simulink model "state_machine"  (R2017b)
settings: Solver=FixedStepAuto  StartTime=0.0  StopTime=1000  FixedStep=0.01  RelTol=1e-3
model workspace (MAT data in the model file):
  SL_ROS_VariableLengthArrays_MaxSizes.CommonInfo.ArrayTruncateAction = 'EmitWarning'
  SL_ROS_VariableLengthArrays_MaxSizes.MsgTypeMap = containers.Map
  SL_ROS_VariableLengthArrays_MaxSizes.MsgTypeMap.serialization.keys = {'sensor_msgs/JointState', 'trajectory_msgs/JointTrajectory', 'trajectory_msgs/JointTrajectoryPoint'}
  SL_ROS_VariableLengthArrays_MaxSizes.MsgTypeMap.serialization.values{1}(1).PropertyName = 'Effort'
  SL_ROS_VariableLengthArrays_MaxSizes.MsgTypeMap.serialization.values{1}(1).DataType = 'double'
  SL_ROS_VariableLengthArrays_MaxSizes.MsgTypeMap.serialization.values{1}(1).MaxLength = 7
  SL_ROS_VariableLengthArrays_MaxSizes.MsgTypeMap.serialization.values{1}(2).PropertyName = 'Name'
  SL_ROS_VariableLengthArrays_MaxSizes.MsgTypeMap.serialization.values{1}(2).DataType = 'std_msgs/String'
  SL_ROS_VariableLengthArrays_MaxSizes.MsgTypeMap.serialization.values{1}(2).MaxLength = 7
  SL_ROS_VariableLengthArrays_MaxSizes.MsgTypeMap.serialization.values{1}(3).PropertyName = 'Position'
  SL_ROS_VariableLengthArrays_MaxSizes.MsgTypeMap.serialization.values{1}(3).DataType = 'double'
  SL_ROS_VariableLengthArrays_MaxSizes.MsgTypeMap.serialization.values{1}(3).MaxLength = 7
  SL_ROS_VariableLengthArrays_MaxSizes.MsgTypeMap.serialization.values{1}(4).PropertyName = 'Velocity'
  SL_ROS_VariableLengthArrays_MaxSizes.MsgTypeMap.serialization.values{1}(4).DataType = 'double'
  SL_ROS_VariableLengthArrays_MaxSizes.MsgTypeMap.serialization.values{1}(4).MaxLength = 7
  SL_ROS_VariableLengthArrays_MaxSizes.MsgTypeMap.serialization.values{2}(1).PropertyName = 'JointNames'
  SL_ROS_VariableLengthArrays_MaxSizes.MsgTypeMap.serialization.values{2}(1).DataType = 'std_msgs/String'
  SL_ROS_VariableLengthArrays_MaxSizes.MsgTypeMap.serialization.values{2}(1).MaxLength = 7
  SL_ROS_VariableLengthArrays_MaxSizes.MsgTypeMap.serialization.values{2}(2).PropertyName = 'Points'
  SL_ROS_VariableLengthArrays_MaxSizes.MsgTypeMap.serialization.values{2}(2).DataType = 'trajectory_msgs/JointTrajectoryPoint'
  SL_ROS_VariableLengthArrays_MaxSizes.MsgTypeMap.serialization.values{2}(2).MaxLength = 1
  SL_ROS_VariableLengthArrays_MaxSizes.MsgTypeMap.serialization.values{3}(1).PropertyName = 'Accelerations'
  SL_ROS_VariableLengthArrays_MaxSizes.MsgTypeMap.serialization.values{3}(1).DataType = 'double'
  SL_ROS_VariableLengthArrays_MaxSizes.MsgTypeMap.serialization.values{3}(1).MaxLength = 7
  SL_ROS_VariableLengthArrays_MaxSizes.MsgTypeMap.serialization.values{3}(2).PropertyName = 'Effort'
  SL_ROS_VariableLengthArrays_MaxSizes.MsgTypeMap.serialization.values{3}(2).DataType = 'double'
  SL_ROS_VariableLengthArrays_MaxSizes.MsgTypeMap.serialization.values{3}(2).MaxLength = 7
  SL_ROS_VariableLengthArrays_MaxSizes.MsgTypeMap.serialization.values{3}(3).PropertyName = 'Positions'
  SL_ROS_VariableLengthArrays_MaxSizes.MsgTypeMap.serialization.values{3}(3).DataType = 'double'
  SL_ROS_VariableLengthArrays_MaxSizes.MsgTypeMap.serialization.values{3}(3).MaxLength = 7
  SL_ROS_VariableLengthArrays_MaxSizes.MsgTypeMap.serialization.values{3}(4).PropertyName = 'Velocities'
  SL_ROS_VariableLengthArrays_MaxSizes.MsgTypeMap.serialization.values{3}(4).DataType = 'double'
  SL_ROS_VariableLengthArrays_MaxSizes.MsgTypeMap.serialization.values{3}(4).MaxLength = 7
  SL_ROS_VariableLengthArrays_MaxSizes.MsgTypeMap.serialization.uniformity = 0
  SL_ROS_VariableLengthArrays_MaxSizes.MsgTypeMap.serialization.keyType = 'char'
  SL_ROS_VariableLengthArrays_MaxSizes.MsgTypeMap.serialization.valueType = 'any'
values from neighbouring files (symbols this model uses):
  pos_threshold = 0.1    [init.m]
  t_prova = [800,800,800]    [init.m]
  wp = [[wp1_pos;wp1_rot],[wp2_pos;wp2_rot], [wp3_pos; wp3_rot]]    [init.m]
undefined symbols (not defined in the file or in its folder): q_0_right
libraries: robotlib x4, realtime_pacer_lib x1
settings Model: Creator=Chiara  LastModifiedBy=Chiara

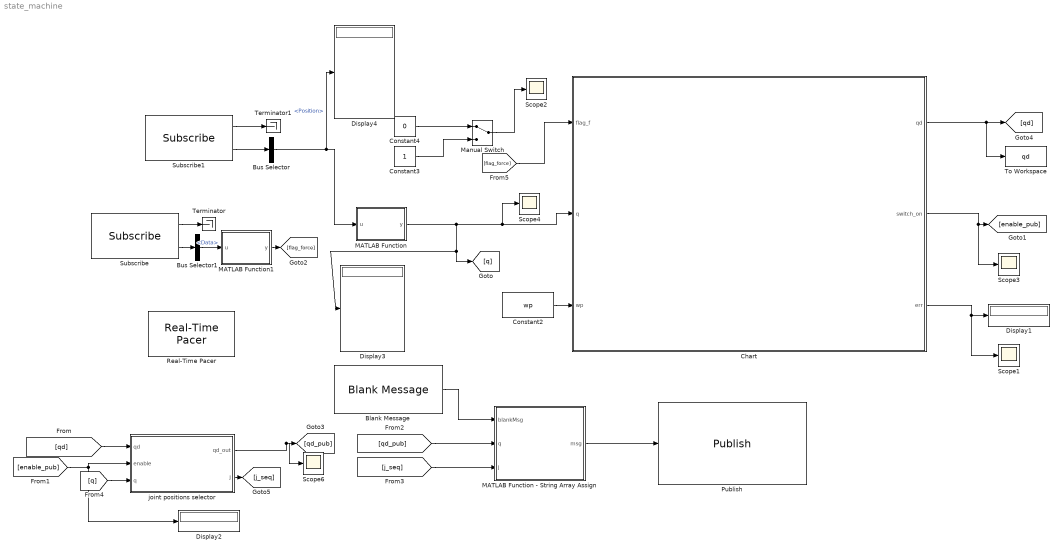
== system state_machine ==
  Blank Message : robotlib/Blank Message  SourceLibraryInfo=This block requires Robotics System Toolbox  messageType=trajectory_msgs/JointTrajectory  SampleTime=-1
      settings: SourceProductBaseCode=RO
  Bus Selector : BusSelector  OutputSignals=Position
  Bus Selector1 : BusSelector  OutputSignals=Data
  Chart : Stateflow chart  TreatAsAtomicUnit=on
  Constant2 : Constant  Value=wp
  Constant3 : Constant
  Constant4 : Constant  Value=0
  Display{1..4} (4 alike) : Display
  MATLAB Function : MATLAB Function  TreatAsAtomicUnit=on
  MATLAB Function - String Array Assign : MATLAB Function  TreatAsAtomicUnit=on
  MATLAB Function1 : MATLAB Function  TreatAsAtomicUnit=on
  Manual Switch : ManualSwitch
  Publish : robotlib/Publish  SourceLibraryInfo=This block requires Robotics System Toolbox  topicSource=Specify your own  topic=/right_arm/joint_trajectory_controller/command_aux  messageType=trajectory_msgs/JointTrajectory  messageQueueLength=1
      settings: SourceProductBaseCode=RO
  Real-Time Pacer : realtime_pacer_lib/Real-Time Pacer  simTimePerRealTime=1
  Scope{1..4,6} (5 alike) : Scope
  Subscribe : robotlib/Subscribe  SourceLibraryInfo=This block requires Robotics System Toolbox  topicSource=Specify your own  topic=/arms_manager/force_flag_right  messageType=std_msgs/Bool  sampleTime=-1  messageQueueLength=1
      settings: SourceProductBaseCode=RO
  Subscribe1 : robotlib/Subscribe  SourceLibraryInfo=This block requires Robotics System Toolbox  topicSource=Specify your own  topic=/right_arm/joint_states  messageType=sensor_msgs/JointState  sampleTime=-1  messageQueueLength=1
      settings: SourceProductBaseCode=RO
  Terminator : Terminator
  Terminator1 : Terminator
  To Workspace : ToWorkspace  VariableName=qd  SaveFormat=Timeseries  SampleTime=-1
  joint positions selector : MATLAB Function  TreatAsAtomicUnit=on
  wires:
  Constant2/1 -> Chart/3(wp)
  [qd] -> joint positions selector/1(qd)
  Chart/1(qd) -> To Workspace/1, [qd]
  Chart/2(switch_on) -> Scope3/1, [enable_pub]
  [enable_pub] -> Display2/1, joint positions selector/2(enable)
  Subscribe/2 -> Bus Selector1/1
  Subscribe/1 -> Terminator/1
  Subscribe1/1 -> Terminator1/1
  Subscribe1/2 -> Bus Selector/1
  Manual Switch/1 -> Scope2/1
  Blank Message/1 -> MATLAB Function - String Array Assign/1(blankMsg)
  MATLAB Function - String Array Assign/1(msg) -> Publish/1
  Constant4/1 -> Manual Switch/1
  Constant3/1 -> Manual Switch/2
  joint positions selector/1(qd_out) -> Scope6/1, [qd_pub]
  [qd_pub] -> MATLAB Function - String Array Assign/2(q)
  joint positions selector/2(j) -> [j_seq]
  [j_seq] -> MATLAB Function - String Array Assign/3(j)
  Bus Selector/1 -> Display4/1, MATLAB Function/1(u)  "<Position>"
  Chart/3(err) -> Scope1/1, Display1/1
  MATLAB Function/1(y) -> Display3/1, [q], Scope4/1, Chart/2(q)
  [q] -> joint positions selector/3(q)
  [flag_force] -> Chart/1(flag_f)
  Bus Selector1/1 -> MATLAB Function1/1(u)  "<Data>"
  MATLAB Function1/1(y) -> [flag_force]

== matlab function state_machine/joint positions selector ==
  data: qd input; enable input; qd_out output; j output; q input
function [qd_out, j] = publisher_(qd, enable, q)
%% 
%qd_out = points to be send to the robot
%qd = entire trajectory generated by reverse priority
% enable = equal to 1 once a trajectpry qd has been generated by rev
% priority
%%
% if qd has been generated, this function selects consecutive joint
% positions along the trajectory qd to be send to the robot
persistent count 

if(isempty(count))
    count=0;
end

qd_out = q';

if( enable == 1 )
   count = count + 1;
   if (count > size(qd,2))
       count =  size(qd,2);
   end
   qd_out = qd(:,count);
else
    count = 0;
end
j = count;
end

== matlab function state_machine/MATLAB Function ==
  data: u input; y output
function y = fcn(u)
y = u';
    y(3) = u(7);
    for i = 4 : 7
       y(i) = u(i-1);
    end

== stateflow chart state_machine/Chart ==
  settings: updateMethod=DISCRETE  sampleTime=0-01
  state state1
    en:
    flag_pos = 0;
    coder.extrinsic('traj_line_0');
    switch_on =0;
    qd_local = traj_line_0(t_prova(1), q_0_right, wp(1:3,1), wp(4:end,1));
    qd = [qd_local, repmat(qd_local(1:7, t_prova(1)) ,1, 1000-t_prova(1))];
    du:
    switch_on = 1;
    err = max(abs(angdiff(qd(:,end),q')));
    if(err <= pos_threshold && err~=0)
    flag_pos = 1;
    end
    ex:
    q_0_ = q';
  state state2
    en: coder.extrinsic('traj_line_');
    switch_on =0;
    qd_local =  traj_line_(t_prova(2), q_0_, wp(1:3,2), wp(4:end,2));
    qd = [qd_local, repmat(qd_local(1:7,t_prova(2)) , 1,1000-t_prova(2))];
    du:
    err = max(abs(angdiff(qd(:,end),q')));
    if(err <= pos_threshold && err~=0)
    flag_pos = 1;
    end
    switch_on = 1;
    ex:
    q_0_ = q';
  state state3
    en: coder.extrinsic('traj_line_');
    switch_on = 0;
    qd_local = traj_line_(t_prova(3), q_0_, wp(1:3,3), wp(4:end,3));
    qd = [qd_local, repmat(qd_local(1:7,t_prova(3)) , 1, 1000-t_prova(3))];
    du:
    err = max(abs(angdiff(qd(:,end),q')));
    if(err <= pos_threshold && err~=0)
    flag_pos = 1;
    end
    switch_on = 1;
    ex:
    q_0_ = q';
  (default) -> state1
  state1 -> state2 : [flag_f == 1||flag_pos ==1]{flag_pos = 0;switch_on =0;}
  state3 -> state2 : [flag_f ==1||flag_pos == 1]{flag_pos = 0;switch_on =0;}
  state2 -> state3 : [flag_f ==1||flag_pos == 1]{flag_pos = 0;switch_on =0;}
  data: qd output double size=[7 1000]; switch_on output; flag_f input; q input; wp input; q_0_ local; qd_ local; pos_threshold parameter; flag_pos local; t_prova parameter; q_0_right parameter; err output; qd_local local

== matlab function state_machine/MATLAB Function1 ==
  data: u input; y output
function y = fcn(u)
persistent u_old
if(isempty(u_old))
    u_old = 0;
end
if(u_old == 0 && u == 1)
    y =1;
else
    y=0;
end

u_old = double(u);

== matlab function state_machine/MATLAB Function - String Array Assign ==
  data: blankMsg input; msg output Bus: SL_Bus_state_machine_trajectory_msgs_JointTrajectory; q input; j input
function msg = stringArrayAssign(blankMsg,q,j)
% stringArrayAssign - Assign a string array in a ROS message
%
%  blankMsg (input): A bus for a 'sensor_msgs/JointState' message. This is 
%      used to initialize the output.
%  msg (output): A bus for a 'sensor_msgs/JointState' message message, with 
%      Name field set to a string array.
%
%   Copyright 2015 The MathWorks, Inc.

%#codegen

% Note: The datatype of 'msg' has been explicitly set to the appropriate 
% Simulink bus type ("SL_Bus_robotROSMessageUsageExample_sensor_msgs_JointState"). 
%
% If the model name is changed, the datatype needs to be changed as well:
%   1) Click "Edit Data" in the Editor toolstrip to open "Ports and Data Manager"
%   2) Select "msg". From the "Type" dropdown, select "--- Refresh data types ---"
%   3) Set datatype to "Bus: SL_Bus_<modelname>_sensor_msgs_JointState"

strArrayToAssign = {'right_arm_a1_joint', 'right_arm_a2_joint', 'right_arm_e1_joint', 'right_arm_a3_joint', 'right_arm_a4_joint', 'right_arm_a5_joint', 'right_arm_a6_joint'};
msg = blankMsg;

% Set the number of strings in the string array.
% msg (sensor_msgs/JointState) includes the following fields
%           Name : array of std_msgs/String (string array)
%   Name_SL_Info : struct with fields CurrentLength, ReceivedLength
numStringsInArray = length(strArrayToAssign);
msg.JointNames_SL_Info.CurrentLength = uint32(numStringsInArray);
msg.Points_SL_Info.CurrentLength = uint32(1);
% Set the individual strings in the array
for idx=1:numStringsInArray
    str = strArrayToAssign{idx};
    strLength = length(str);
    msg.JointNames(idx).Data(1:strLength) = uint8(str);
    msg.JointNames(idx).Data_SL_Info.CurrentLength = uint32(strLength);
end
msg.Points(1).Positions(1:length(q)) = q;
msg.Points(1).Positions_SL_Info.CurrentLength = uint32(length(q));
msg.Points(1).TimeFromStart.Sec = 0;
msg.Points(1).TimeFromStart.Nsec = 5000000;

msg.Header.Seq = uint32(j);
